simulink model "CM670A_HwAg1Meas"  (R2013b)
settings: Solver=FixedStepDiscrete  SolverMode=SingleTasking  StartTime=0.0  StopTime=22  FixedStep=0.002  RelTol=1e-3
values from neighbouring files (symbols this model uses):
  ELECGLBPRM_DEGPERREV_DEGPERREV_F32 = DataDict.Constant    [CM670A_HwAg1Meas_DataDict.m]
  ELECGLBPRM_HWAGCENTROFFS_HWDEG_F32 = DataDict.Constant    [CM670A_HwAg1Meas_DataDict.m]
  ELECGLBPRM_HWAGSATNLOWRLIM_HWDEG_F32 = DataDict.Constant    [CM670A_HwAg1Meas_DataDict.m]
  ELECGLBPRM_HWAGSATNUPPRLIM_HWDEG_F32 = DataDict.Constant    [CM670A_HwAg1Meas_DataDict.m]
  ELECGLBPRM_HWAGSCA_ULS_F32 = DataDict.Constant    [CM670A_HwAg1Meas_DataDict.m]
  ELECGLBPRM_HWAGSPURGEARRAT_ULS_F32 = DataDict.Constant    [CM670A_HwAg1Meas_DataDict.m]
  ELECGLBPRM_HWAGSPURTORINGGEARRATSNSR0_ULS_F32 = DataDict.Constant    [CM670A_HwAg1Meas_DataDict.m]
  ELECGLBPRM_HWAGSPURTORINGGEARRATSNSR1_ULS_F32 = DataDict.Constant    [CM670A_HwAg1Meas_DataDict.m]
  ELECGLBPRM_NOFLT_CNT_U08 = DataDict.Constant    [CM670A_HwAg1Meas_DataDict.m]
  ELECGLBPRM_OFFSTRIMNOTPRFMD_CNT_U08 = DataDict.Constant    [CM670A_HwAg1Meas_DataDict.m]
  ELECGLBPRM_PRTCLFLT_CNT_U08 = DataDict.Constant    [CM670A_HwAg1Meas_DataDict.m]
  ELECGLBPRM_SKIPSTEPFLT_CNT_U08 = DataDict.Constant    [CM670A_HwAg1Meas_DataDict.m]
  ELECGLBPRM_SNSRINTFLT_CNT_U08 = DataDict.Constant    [CM670A_HwAg1Meas_DataDict.m]
  ELECGLBPRM_VRNRERRFLT_CNT_U08 = DataDict.Constant    [CM670A_HwAg1Meas_DataDict.m]
  HWAG10THTOOTHTRIG_CNT_U08 = DataDict.ConfigParam    [CM670A_HwAg1Meas_DataDict.m]
  HWAG11THTOOTHTRIG_CNT_U08 = DataDict.ConfigParam    [CM670A_HwAg1Meas_DataDict.m]
  HwAg1IfFlt = DataDict.NTC    [CM670A_HwAg1Meas_DataDict.m]
  HwAg1MeasHwAg1IfFltFailStep = DataDict.Calibration    [CM670A_HwAg1Meas_DataDict.m]
  HwAg1MeasHwAg1IfFltPassStep = DataDict.Calibration    [CM670A_HwAg1Meas_DataDict.m]
  HwAg1MeasHwAg1Snsr0PrtclFltFailStep = DataDict.Calibration    [CM670A_HwAg1Meas_DataDict.m]
  HwAg1MeasHwAg1Snsr0PrtclFltPassStep = DataDict.Calibration    [CM670A_HwAg1Meas_DataDict.m]
  HwAg1MeasHwAg1Snsr1PrtclFltFailStep = DataDict.Calibration    [CM670A_HwAg1Meas_DataDict.m]
  HwAg1MeasHwAg1Snsr1PrtclFltPassStep = DataDict.Calibration    [CM670A_HwAg1Meas_DataDict.m]
  HwAg1MeasSnsr0Rev = DataDict.Calibration    [CM670A_HwAg1Meas_DataDict.m]
  HwAg1MeasSnsr1Rev = DataDict.Calibration    [CM670A_HwAg1Meas_DataDict.m]
  HwAg1MeasStep = DataDict.Calibration    [CM670A_HwAg1Meas_DataDict.m]
  HwAg1MeasVrnrErrThd = DataDict.Calibration    [CM670A_HwAg1Meas_DataDict.m]
  HwAg1MfgFlt = DataDict.NTC    [CM670A_HwAg1Meas_DataDict.m]
  HwAg1Snsr0PrtclFlt = DataDict.NTC    [CM670A_HwAg1Meas_DataDict.m]
  HwAg1Snsr1PrtclFlt = DataDict.NTC    [CM670A_HwAg1Meas_DataDict.m]
undefined symbols (not defined in the file or in its folder): NtcSts1, sigbuilder_block, SigQlfr1
libraries: simulink x30, NxtrNvM x3
(part 3 of 5)

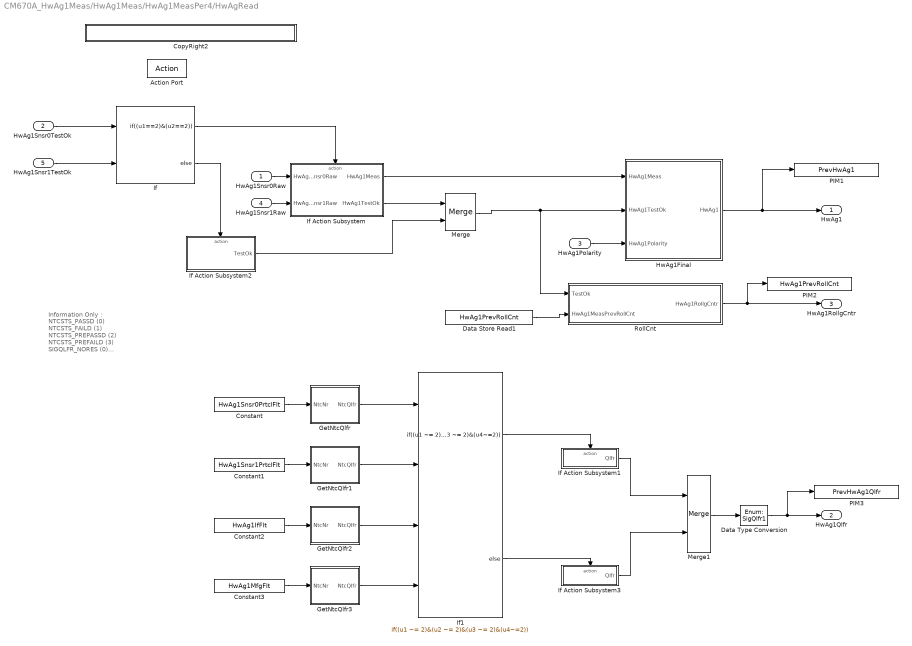
== system CM670A_HwAg1Meas/HwAg1Meas/HwAg1MeasPer4/HwAgRead ==
  note: Information Only :
      |
      | NTCSTS_PASSD            (0)
      | NTCSTS_FAILD              (1)
      | NTCSTS_PREPASSD    (2)
      | NTCSTS_PREFAILD      (3)
      |
      | SIGQLFR_NORES         (0)
      | SIGQLFR_PASSD          (1)
      | SIGQLFR_FAILD            (2)
  HwAg1Snsr0Raw : Inport
  HwAg1Snsr0TestOk : Inport  Port=2
  HwAg1Polarity : Inport  Port=3
  HwAg1Snsr1Raw : Inport  Port=4
  HwAg1Snsr1TestOk : Inport  Port=5
  Action Port : ActionPort  ActionType=then
  Constant : Constant  Value=HwAg1Snsr0PrtclFlt
  Constant1 : Constant  Value=HwAg1Snsr1PrtclFlt
  Constant2 : Constant  Value=HwAg1IfFlt
  Constant3 : Constant  Value=HwAg1MfgFlt
  CopyRight2 : Subsystem  Description=|  mask(Copyright Information){none=on}
      | Copyright info block.                                               
      |                                                                     
      | Place copyright information at the top of every subsystem in design.
      mask prompts: none "No parameters"
      mask help: Place copyright information at the top of every subsystem in design.
      mask Display:
      | NxtrConf = 'Nexteer Confidential';
      | 
      | sys = bdroot; %handle for the current model ("system")
      | first = get_param(sys,'Created');
      | first = first(end-3:end);  %year is last four digits
      | 
      | last = get_param(sys,'LastModifiedDate');
      | if isempty(last)
      |     last = datestr(now,'yyyy');
      | else
      |     last = last(end-3:end);
      | end
      | 
      | if strcmp(first,last)
      |     fprintf('%s -- Copyright %s Nexteer',NxtrConf,first)
      | else
      |     fprintf('%s -- %s%s- %s Nexteer',NxtrConf,char(169),first,last)
      | end
  Data Store Read1 : DataStoreRead  Priority=1  DataStoreName=HwAg1PrevRollCnt
  Data Type Conversion : DataTypeConversion  OutDataTypeStr=Enum: SigQlfr1
  GetNtcQlfr : Subsystem
  GetNtcQlfr1 : Subsystem
  GetNtcQlfr2 : Subsystem
  GetNtcQlfr3 : Subsystem
  HwAg1Final : Subsystem  RequirementInfo={'linktype_rmi_doors' '0000cf44 (/ESG Group/FDD Module Requirements/EA4 Specific/CM670A_HwAg1Meas)' '#CM670A_29' 'true' 'REQ: CM670A_29' '' ; 'linktype_rmi_doors' '0000cf44 (/ESG Group/FDD Module Requirements/EA4 Specific/CM670A_HwAg1Meas)' '#CM670A_32' 'true' 'REQ: CM670A_32' '' ; 'linktype_rmi_doors' '0000cf44 (/ESG Group/FDD Module Requirements/EA4 Specific/CM670A_HwAg1Meas)' '#CM670A_33' 'true' 'REQ: CM670A_33' '' } %GIDa_390fff4e_e0e4_4e0a_b1c2_f884cd2ad424
  If : If  NumInputs=2  IfExpression=(u1==2)&(u2==2)
  If Action Subsystem : Subsystem  TreatAsAtomicUnit=on
  If Action Subsystem1 : Subsystem  TreatAsAtomicUnit=on
  If Action Subsystem2 : Subsystem  TreatAsAtomicUnit=on
  If Action Subsystem3 : Subsystem  TreatAsAtomicUnit=on
  If1 : If  NumInputs=4  IfExpression=(u1 ~= 2)&(u2 ~= 2)&(u3 ~= 2)&(u4~=2)
  Merge : Merge
  Merge1 : Merge
  PIM1 : DataStoreWrite  RequirementInfo={} %GIDa_84bafa65_5fe1_4ee7_b90d_66bb4b4a2750  DataStoreName=PrevHwAg1
  PIM2 : DataStoreWrite  RequirementInfo={} %GIDa_617928b4_a9d1_4855_8092_551055b61714  Priority=2  DataStoreName=HwAg1PrevRollCnt
  PIM3 : DataStoreWrite  RequirementInfo={} %GIDa_3e11a627_fc39_44fa_9faf_fc285a087ff6  DataStoreName=PrevHwAg1Qlfr
  RollCnt : Stateflow chart  RequirementInfo={} %GIDa_3031df54_87b3_4189_88b6_56458e12ea75  TreatAsAtomicUnit=on
  HwAg1 : Outport  RequirementInfo={} %GIDa_c23b8355_c0ea_454a_a0f8_21e7eda4151f
  HwAg1Qlfr : Outport  RequirementInfo={'linktype_rmi_doors' '0000cf44 (/ESG Group/FDD Module Requirements/EA4 Specific/CM670A_HwAg1Meas)' '#CM670A_30' 'true' 'REQ: CM670A_30' '' } %GIDa_9c26b5fb_6b25_41c5_ba2e_96f197c0dca5  Port=2
  HwAg1RollgCntr : Outport  RequirementInfo={'linktype_rmi_doors' '0000cf44 (/ESG Group/FDD Module Requirements/EA4 Specific/CM670A_HwAg1Meas)' '#CM670A_31' 'true' 'REQ: CM670A_31' '' } %GIDa_eb7690db_9bf5_403e_b0dd_c189c54068be  Port=3
  wires:
  RollCnt/1(HwAg1RollgCntr) -> PIM2/1, HwAg1RollgCntr/1
  Constant/1 -> GetNtcQlfr/1(NtcNr)
  HwAg1Snsr0TestOk/1 -> If/1
  HwAg1Snsr1TestOk/1 -> If/2
  If/1 -> If Action Subsystem/Action
  If/2 -> If Action Subsystem2/Action
  If Action Subsystem2/1(TestOk) -> Merge/2
  If Action Subsystem/1(HwAg1Meas) -> HwAg1Final/1(HwAg1Meas)
  Constant1/1 -> GetNtcQlfr1/1(NtcNr)
  Constant2/1 -> GetNtcQlfr2/1(NtcNr)
  GetNtcQlfr/1(NtcQlfr) -> If1/1
  GetNtcQlfr1/1(NtcQlfr) -> If1/2
  GetNtcQlfr2/1(NtcQlfr) -> If1/3
  If1/1 -> If Action Subsystem1/Action
  If1/2 -> If Action Subsystem3/Action
  Merge1/1 -> Data Type Conversion/1
  If Action Subsystem1/1(Qlfr) -> Merge1/1
  If Action Subsystem3/1(Qlfr) -> Merge1/2
  If Action Subsystem/2(HwAg1TestOk) -> Merge/1
  HwAg1Polarity/1 -> HwAg1Final/3(HwAg1Polarity)
  GetNtcQlfr3/1(NtcQlfr) -> If1/4
  Constant3/1 -> GetNtcQlfr3/1(NtcNr)
  Merge/1 -> HwAg1Final/2(HwAg1TestOk), RollCnt/1(TestOk)
  HwAg1Final/1(HwAg1) -> PIM1/1, HwAg1/1
  HwAg1Snsr0Raw/1 -> If Action Subsystem/1(HwAg1Snsr0Raw)
  HwAg1Snsr1Raw/1 -> If Action Subsystem/2(HwAg1Snsr1Raw)
  Data Store Read1/1 -> RollCnt/2(HwAg1MeasPrevRollCnt)
  Data Type Conversion/1 -> PIM3/1, HwAg1Qlfr/1

== system CM670A_HwAg1Meas/HwAg1Meas/HwAg1MeasPer5/CopyRight2 ==

== system CM670A_HwAg1Meas/HwAg1Meas/HwAg1MeasPer5/If Action Subsystem ==
  Action Port : ActionPort  ActionType=then
  CopyRight2 : Subsystem  Description=|  mask(Copyright Information){none=on}
      | Copyright info block.                                               
      |                                                                     
      | Place copyright information at the top of every subsystem in design.
      mask prompts: none "No parameters"
      mask help: Place copyright information at the top of every subsystem in design.
      mask Display:
      | NxtrConf = 'Nexteer Confidential';
      | 
      | sys = bdroot; %handle for the current model ("system")
      | first = get_param(sys,'Created');
      | first = first(end-3:end);  %year is last four digits
      | 
      | last = get_param(sys,'LastModifiedDate');
      | if isempty(last)
      |     last = datestr(now,'yyyy');
      | else
      |     last = last(end-3:end);
      | end
      | 
      | if strcmp(first,last)
      |     fprintf('%s -- Copyright %s Nexteer',NxtrConf,first)
      | else
      |     fprintf('%s -- %s%s- %s Nexteer',NxtrConf,char(169),first,last)
      | end
  Data Type Conversion : DataTypeConversion  OutDataTypeStr=uint8
  NoFlt : Constant  RequirementInfo={} %GIDa_af25b43f_e757_49bd_94aa_be1229c5c8b6  Value=ELECGLBPRM_NOFLT_CNT_U08  OutDataTypeStr=uint8
  NtcSts : simulink/Sources/Enumerated Constant  OutDataTypeStr=Enum: NtcSts1  Value=NtcSts1.NTCSTS_PASSD  SampleTime=inf
  ParamByte : Outport
  TestOk : Outport  Port=2
  wires:
  NtcSts/1 -> Data Type Conversion/1
  NoFlt/1 -> ParamByte/1
  Data Type Conversion/1 -> TestOk/1

== system CM670A_HwAg1Meas/HwAg1Meas/HwAg1MeasPer5/If Action Subsystem1 ==
  Action Port : ActionPort  ActionType=else
  CopyRight2 : Subsystem  Description=|  mask(Copyright Information){none=on}
      | Copyright info block.                                               
      |                                                                     
      | Place copyright information at the top of every subsystem in design.
      mask prompts: none "No parameters"
      mask help: Place copyright information at the top of every subsystem in design.
      mask Display:
      | NxtrConf = 'Nexteer Confidential';
      | 
      | sys = bdroot; %handle for the current model ("system")
      | first = get_param(sys,'Created');
      | first = first(end-3:end);  %year is last four digits
      | 
      | last = get_param(sys,'LastModifiedDate');
      | if isempty(last)
      |     last = datestr(now,'yyyy');
      | else
      |     last = last(end-3:end);
      | end
      | 
      | if strcmp(first,last)
      |     fprintf('%s -- Copyright %s Nexteer',NxtrConf,first)
      | else
      |     fprintf('%s -- %s%s- %s Nexteer',NxtrConf,char(169),first,last)
      | end
  Data Type Conversion : DataTypeConversion  OutDataTypeStr=uint8
  NoFlt : Constant  RequirementInfo={} %GIDa_a79c1974_b7e9_4639_b05c_c7a17ce1d256  Value=ELECGLBPRM_OFFSTRIMNOTPRFMD_CNT_U08  OutDataTypeStr=uint8
  NtcSts : simulink/Sources/Enumerated Constant  OutDataTypeStr=Enum: NtcSts1  Value=NtcSts1.NTCSTS_FAILD  SampleTime=inf
  ParamByte : Outport
  TestOk : Outport  Port=2
  wires:
  NoFlt/1 -> ParamByte/1
  NtcSts/1 -> Data Type Conversion/1
  Data Type Conversion/1 -> TestOk/1

== system CM670A_HwAg1Meas/HwAg1Meas/HwAg1MeasPer5/SetNtcSts ==
  note: Note:
      |
      | - "ISO Fault Debounce Design" Simulink block intent to use here for Simulation purpose only. Do not Code this block
  NtcNr : Inport
  NtcStInfo : Inport  Port=2
  NtcSts : Inport  Port=3
  DebStep : Inport  Port=4
  CopyRight2 : Subsystem  Description=|  mask(Copyright Information){none=on}
      | Copyright info block.                                               
      |                                                                     
      | Place copyright information at the top of every subsystem in design.
      mask prompts: none "No parameters"
      mask help: Place copyright information at the top of every subsystem in design.
      mask Display:
      | NxtrConf = 'Nexteer Confidential';
      | 
      | sys = bdroot; %handle for the current model ("system")
      | first = get_param(sys,'Created');
      | first = first(end-3:end);  %year is last four digits
      | 
      | last = get_param(sys,'LastModifiedDate');
      | if isempty(last)
      |     last = datestr(now,'yyyy');
      | else
      |     last = last(end-3:end);
      | end
      | 
      | if strcmp(first,last)
      |     fprintf('%s -- Copyright %s Nexteer',NxtrConf,first)
      | else
      |     fprintf('%s -- %s%s- %s Nexteer',NxtrConf,char(169),first,last)
      | end
  Data Store Write : DataStoreWrite  DataStoreName=Ntc0X1FAQlfr
  Ground : Ground
  ISO Fault Debounce Design : Stateflow chart  TreatAsAtomicUnit=on
      settings: AttributesFormatString=|
      | Simulation Purpose Only.
      | Do Not Code this block
      | Diagnostic Manager Owns this requirement
  Scope1 : Scope  NumInputPorts=3
      settings: YMin=-5~-5~-5  YMax=5~5~5  SaveName=ScopeData5
  Terminator : Terminator
  Terminator1 : Terminator
  wires:
  Ground/1 -> ISO Fault Debounce Design/3(SvcClr)
  ISO Fault Debounce Design/1(Qualifier) -> Data Store Write/1, Scope1/3
  DebStep/1 -> Scope1/2, ISO Fault Debounce Design/2(DebStep)
  NtcSts/1 -> Scope1/1, ISO Fault Debounce Design/1(NtcSts)
  NtcNr/1 -> Terminator/1
  NtcStInfo/1 -> Terminator1/1

== system CM670A_HwAg1Meas/HwAg1Meas/HwAg1MeasInit1/GetRefTmr1MicroSec32bit/CopyRight2 ==

== system CM670A_HwAg1Meas/HwAg1Meas/HwAg1MeasInit1/GetTiSpan1MicroSec32bit/CopyRight2 ==

== system CM670A_HwAg1Meas/HwAg1Meas/HwAg1MeasInit1/IoHwAb_SetFctPrphlHwAg1/CopyRight2 ==

== system CM670A_HwAg1Meas/HwAg1Meas/HwAg1MeasPer1/GetRefTmr1MicroSec32bit1/CopyRight2 ==

== system CM670A_HwAg1Meas/HwAg1Meas/HwAg1MeasPer1/GetTiSpan1MicroSec32bit/CopyRight2 ==

== system CM670A_HwAg1Meas/HwAg1Meas/HwAg1MeasPer1/IncrementCount/CopyRight2 ==

== system CM670A_HwAg1Meas/HwAg1Meas/HwAg1MeasPer1/ResetCount/CopyRight2 ==

== system CM670A_HwAg1Meas/HwAg1Meas/HwAg1MeasPer2/Snsr0Read/CopyRight2 ==

== system CM670A_HwAg1Meas/HwAg1Meas/HwAg1MeasPer2/Snsr0Read/DebStepSelection ==
  TestOk : Inport
  CopyRight2 : Subsystem  Description=|  mask(Copyright Information){none=on}
      | Copyright info block.                                               
      |                                                                     
      | Place copyright information at the top of every subsystem in design.
      mask prompts: none "No parameters"
      mask help: Place copyright information at the top of every subsystem in design.
      mask Display:
      | NxtrConf = 'Nexteer Confidential';
      | 
      | sys = bdroot; %handle for the current model ("system")
      | first = get_param(sys,'Created');
      | first = first(end-3:end);  %year is last four digits
      | 
      | last = get_param(sys,'LastModifiedDate');
      | if isempty(last)
      |     last = datestr(now,'yyyy');
      | else
      |     last = last(end-3:end);
      | end
      | 
      | if strcmp(first,last)
      |     fprintf('%s -- Copyright %s Nexteer',NxtrConf,first)
      | else
      |     fprintf('%s -- %s%s- %s Nexteer',NxtrConf,char(169),first,last)
      | end
  NTCFailStepCal : Constant  Value=HwAg1MeasHwAg1Snsr0PrtclFltFailStep
  NTCPassStepCal : Constant  Value=HwAg1MeasHwAg1Snsr0PrtclFltPassStep
  Switch : Switch  Criteria=u2 > Threshold  Threshold=2
  DebStep : Outport  OutDataTypeStr=uint16
  wires:
  NTCFailStepCal/1 -> Switch/1
  Switch/1 -> DebStep/1
  NTCPassStepCal/1 -> Switch/3
  TestOk/1 -> Switch/2

== system CM670A_HwAg1Meas/HwAg1Meas/HwAg1MeasPer2/Snsr0Read/Do nothing ==
  Action Port : ActionPort  ActionType=else
  CopyRight2 : Subsystem  Description=|  mask(Copyright Information){none=on}
      | Copyright info block.                                               
      |                                                                     
      | Place copyright information at the top of every subsystem in design.
      mask prompts: none "No parameters"
      mask help: Place copyright information at the top of every subsystem in design.
      mask Display:
      | NxtrConf = 'Nexteer Confidential';
      | 
      | sys = bdroot; %handle for the current model ("system")
      | first = get_param(sys,'Created');
      | first = first(end-3:end);  %year is last four digits
      | 
      | last = get_param(sys,'LastModifiedDate');
      | if isempty(last)
      |     last = datestr(now,'yyyy');
      | else
      |     last = last(end-3:end);
      | end
      | 
      | if strcmp(first,last)
      |     fprintf('%s -- Copyright %s Nexteer',NxtrConf,first)
      | else
      |     fprintf('%s -- %s%s- %s Nexteer',NxtrConf,char(169),first,last)
      | end

== system CM670A_HwAg1Meas/HwAg1Meas/HwAg1MeasPer2/Snsr0Read/RawHwAgRead ==
  Snsr0CS : Inport
  Snsr0FRS : Inport  Port=2
  Snsr0FCCN : Inport  Port=3
  Snsr0Data : Inport  Port=4
  Snsr0Id : Inport  Port=5
  Bus Selector : BusSelector  OutputSignals=RawHwAg,TestOk,ParamByte
  Bus Selector1 : BusSelector  OutputSignals=RawHwAg,TestOk,ParamByte
  CopyRight2 : Subsystem  Description=|  mask(Copyright Information){none=on}
      | Copyright info block.                                               
      |                                                                     
      | Place copyright information at the top of every subsystem in design.
      mask prompts: none "No parameters"
      mask help: Place copyright information at the top of every subsystem in design.
      mask Display:
      | NxtrConf = 'Nexteer Confidential';
      | 
      | sys = bdroot; %handle for the current model ("system")
      | first = get_param(sys,'Created');
      | first = first(end-3:end);  %year is last four digits
      | 
      | last = get_param(sys,'LastModifiedDate');
      | if isempty(last)
      |     last = datestr(now,'yyyy');
      | else
      |     last = last(end-3:end);
      | end
      | 
      | if strcmp(first,last)
      |     fprintf('%s -- Copyright %s Nexteer',NxtrConf,first)
      | else
      |     fprintf('%s -- %s%s- %s Nexteer',NxtrConf,char(169),first,last)
      | end
  If : If  RequirementInfo={} %GIDa_2f644cf5_4c0f_42f4_aa5e_d14eb49d3684  IfExpression=u1 ~= 0
  Merge : Merge
  Merge1 : Merge
  Merge2 : Merge
  NewMsg : Subsystem  TreatAsAtomicUnit=on
  NoNewMsg : Subsystem  RequirementInfo={'linktype_rmi_doors' '0000cf44 (/ESG Group/FDD Module Requirements/EA4 Specific/CM670A_HwAg1Meas)' '#CM670A_47' 'true' 'REQ: CM670A_47' '' } %GIDa_69e0972d_6120_427f_87c3_f6166b66255c  TreatAsAtomicUnit=on
      mask Display: disp('NoNewMsg')
  Snsr0Scope : Scope  NumInputPorts=3
      settings: TimeRange=10  YMin=0~1.5~-0.5  YMax=5000~3.5~4.5
  RawHwAg : Outport
  TestOk : Outport  Port=2
  ParamByte : Outport  Port=3
  wires:
  If/1 -> NewMsg/Action  "NoFault"
  If/2 -> NoNewMsg/Action  "Fault"
  NewMsg/1(Out1) -> Bus Selector/1
  NoNewMsg/1(Out1) -> Bus Selector1/1
  Bus Selector1/1 -> Merge2/1  "<RawHwAg>"
  Bus Selector/1 -> Merge2/2  "<RawHwAg>"
  Bus Selector1/2 -> Merge/1  "<TestOk>"
  Bus Selector/2 -> Merge/2  "<TestOk>"
  Bus Selector1/3 -> Merge1/1  "<ParamByte>"
  Bus Selector/3 -> Merge1/2  "<ParamByte>"
  Merge2/1 -> RawHwAg/1, Snsr0Scope/1  "RawHwAg"
  Merge/1 -> Snsr0Scope/2, TestOk/1  "TestOk"
  Merge1/1 -> Snsr0Scope/3, ParamByte/1  "ParamByte"
  Snsr0FRS/1 -> If/1
  Snsr0CS/1 -> NewMsg/1(Snsr0CS)
  Snsr0FCCN/1 -> NewMsg/2(Snsr0FCCN)
  Snsr0Data/1 -> NewMsg/4(Snsr0Data)
  Snsr0Id/1 -> NewMsg/3(Snsr0Id)

== system CM670A_HwAg1Meas/HwAg1Meas/HwAg1MeasPer2/Snsr0Read/Read the Flag ==
  RegInpRSENT2FND : Inport
  Action Port : ActionPort  ActionType=then
  CopyRight2 : Subsystem  Description=|  mask(Copyright Information){none=on}
      | Copyright info block.                                               
      |                                                                     
      | Place copyright information at the top of every subsystem in design.
      mask prompts: none "No parameters"
      mask help: Place copyright information at the top of every subsystem in design.
      mask Display:
      | NxtrConf = 'Nexteer Confidential';
      | 
      | sys = bdroot; %handle for the current model ("system")
      | first = get_param(sys,'Created');
      | first = first(end-3:end);  %year is last four digits
      | 
      | last = get_param(sys,'LastModifiedDate');
      | if isempty(last)
      |     last = datestr(now,'yyyy');
      | else
      |     last = last(end-3:end);
      | end
      | 
      | if strcmp(first,last)
      |     fprintf('%s -- Copyright %s Nexteer',NxtrConf,first)
      | else
      |     fprintf('%s -- %s%s- %s Nexteer',NxtrConf,char(169),first,last)
      | end
  RSENT2DummyRead : Terminator
  wires:
  RegInpRSENT2FND/1 -> RSENT2DummyRead/1

== system CM670A_HwAg1Meas/HwAg1Meas/HwAg1MeasPer2/Snsr0Read/SetNtcSts ==
  note: Note:
      |
      | - "ISO Fault Debounce Design" Simulink block intent to use here for Simulation purpose only. Do not Code this block
  NtcNr : Inport
  NtcStInfo : Inport  Port=2
  NtcSts : Inport  Port=3
  DebStep : Inport  Port=4
  CopyRight2 : Subsystem  Description=|  mask(Copyright Information){none=on}
      | Copyright info block.                                               
      |                                                                     
      | Place copyright information at the top of every subsystem in design.
      mask prompts: none "No parameters"
      mask help: Place copyright information at the top of every subsystem in design.
      mask Display:
      | NxtrConf = 'Nexteer Confidential';
      | 
      | sys = bdroot; %handle for the current model ("system")
      | first = get_param(sys,'Created');
      | first = first(end-3:end);  %year is last four digits
      | 
      | last = get_param(sys,'LastModifiedDate');
      | if isempty(last)
      |     last = datestr(now,'yyyy');
      | else
      |     last = last(end-3:end);
      | end
      | 
      | if strcmp(first,last)
      |     fprintf('%s -- Copyright %s Nexteer',NxtrConf,first)
      | else
      |     fprintf('%s -- %s%s- %s Nexteer',NxtrConf,char(169),first,last)
      | end
  Data Store Write : DataStoreWrite  DataStoreName=Ntc0x097Qlfr
  Ground : Ground
  ISO Fault Debounce Design : Stateflow chart  TreatAsAtomicUnit=on
      settings: AttributesFormatString=|
      | Simulation Purpose Only.
      | Do Not Code this block
      | Diagnostic Manager Owns this requirement
  Scope1 : Scope  NumInputPorts=3
      settings: YMin=-5~-5~-5  YMax=5~5~5  SaveName=ScopeData5
  Terminator : Terminator
  Terminator1 : Terminator
  wires:
  Ground/1 -> ISO Fault Debounce Design/3(SvcClr)
  ISO Fault Debounce Design/1(Qualifier) -> Data Store Write/1, Scope1/3
  DebStep/1 -> Scope1/2, ISO Fault Debounce Design/2(DebStep)
  NtcSts/1 -> Scope1/1, ISO Fault Debounce Design/1(NtcSts)
  NtcNr/1 -> Terminator/1
  NtcStInfo/1 -> Terminator1/1

== system CM670A_HwAg1Meas/HwAg1Meas/HwAg1MeasPer2/Snsr0Read1/CopyRight2 ==

== system CM670A_HwAg1Meas/HwAg1Meas/HwAg1MeasPer3/Snsr1Read/CopyRight2 ==

== system CM670A_HwAg1Meas/HwAg1Meas/HwAg1MeasPer3/Snsr1Read/DebStepSelection ==
  TestOk : Inport
  CopyRight2 : Subsystem  Description=|  mask(Copyright Information){none=on}
      | Copyright info block.                                               
      |                                                                     
      | Place copyright information at the top of every subsystem in design.
      mask prompts: none "No parameters"
      mask help: Place copyright information at the top of every subsystem in design.
      mask Display:
      | NxtrConf = 'Nexteer Confidential';
      | 
      | sys = bdroot; %handle for the current model ("system")
      | first = get_param(sys,'Created');
      | first = first(end-3:end);  %year is last four digits
      | 
      | last = get_param(sys,'LastModifiedDate');
      | if isempty(last)
      |     last = datestr(now,'yyyy');
      | else
      |     last = last(end-3:end);
      | end
      | 
      | if strcmp(first,last)
      |     fprintf('%s -- Copyright %s Nexteer',NxtrConf,first)
      | else
      |     fprintf('%s -- %s%s- %s Nexteer',NxtrConf,char(169),first,last)
      | end
  NTCFailStepCal : Constant  Value=HwAg1MeasHwAg1Snsr1PrtclFltFailStep
  NTCPassStepCal : Constant  Value=HwAg1MeasHwAg1Snsr1PrtclFltPassStep
  Switch : Switch  Criteria=u2 > Threshold  Threshold=2
  DebStep : Outport  OutDataTypeStr=uint16
  wires:
  NTCFailStepCal/1 -> Switch/1
  Switch/1 -> DebStep/1
  NTCPassStepCal/1 -> Switch/3
  TestOk/1 -> Switch/2

== system CM670A_HwAg1Meas/HwAg1Meas/HwAg1MeasPer3/Snsr1Read/Do nothing ==
  Action Port : ActionPort  ActionType=else
  CopyRight2 : Subsystem  Description=|  mask(Copyright Information){none=on}
      | Copyright info block.                                               
      |                                                                     
      | Place copyright information at the top of every subsystem in design.
      mask prompts: none "No parameters"
      mask help: Place copyright information at the top of every subsystem in design.
      mask Display:
      | NxtrConf = 'Nexteer Confidential';
      | 
      | sys = bdroot; %handle for the current model ("system")
      | first = get_param(sys,'Created');
      | first = first(end-3:end);  %year is last four digits
      | 
      | last = get_param(sys,'LastModifiedDate');
      | if isempty(last)
      |     last = datestr(now,'yyyy');
      | else
      |     last = last(end-3:end);
      | end
      | 
      | if strcmp(first,last)
      |     fprintf('%s -- Copyright %s Nexteer',NxtrConf,first)
      | else
      |     fprintf('%s -- %s%s- %s Nexteer',NxtrConf,char(169),first,last)
      | end

== system CM670A_HwAg1Meas/HwAg1Meas/HwAg1MeasPer3/Snsr1Read/Do nothing1 ==
  Action Port : ActionPort  ActionType=else
  CopyRight2 : Subsystem  Description=|  mask(Copyright Information){none=on}
      | Copyright info block.                                               
      |                                                                     
      | Place copyright information at the top of every subsystem in design.
      mask prompts: none "No parameters"
      mask help: Place copyright information at the top of every subsystem in design.
      mask Display:
      | NxtrConf = 'Nexteer Confidential';
      | 
      | sys = bdroot; %handle for the current model ("system")
      | first = get_param(sys,'Created');
      | first = first(end-3:end);  %year is last four digits
      | 
      | last = get_param(sys,'LastModifiedDate');
      | if isempty(last)
      |     last = datestr(now,'yyyy');
      | else
      |     last = last(end-3:end);
      | end
      | 
      | if strcmp(first,last)
      |     fprintf('%s -- Copyright %s Nexteer',NxtrConf,first)
      | else
      |     fprintf('%s -- %s%s- %s Nexteer',NxtrConf,char(169),first,last)
      | end

== system CM670A_HwAg1Meas/HwAg1Meas/HwAg1MeasPer3/Snsr1Read/RawHwAgRead ==
  Snsr1CS : Inport
  Snsr1FRS : Inport  Port=2
  Snsr1FCCN : Inport  Port=3
  Snsr1Data : Inport  Port=4
  Snsr1Id : Inport  Port=5
  Bus Selector : BusSelector  OutputSignals=RawHwAg,TestOk,ParamByte
  Bus Selector1 : BusSelector  OutputSignals=RawHwAg,TestOk,ParamByte
  CopyRight2 : Subsystem  Description=|  mask(Copyright Information){none=on}
      | Copyright info block.                                               
      |                                                                     
      | Place copyright information at the top of every subsystem in design.
      mask prompts: none "No parameters"
      mask help: Place copyright information at the top of every subsystem in design.
      mask Display:
      | NxtrConf = 'Nexteer Confidential';
      | 
      | sys = bdroot; %handle for the current model ("system")
      | first = get_param(sys,'Created');
      | first = first(end-3:end);  %year is last four digits
      | 
      | last = get_param(sys,'LastModifiedDate');
      | if isempty(last)
      |     last = datestr(now,'yyyy');
      | else
      |     last = last(end-3:end);
      | end
      | 
      | if strcmp(first,last)
      |     fprintf('%s -- Copyright %s Nexteer',NxtrConf,first)
      | else
      |     fprintf('%s -- %s%s- %s Nexteer',NxtrConf,char(169),first,last)
      | end
  If : If  RequirementInfo={} %GIDa_15f483e9_befa_45a2_b74e_1f3bb1cc8902  IfExpression=u1 ~= 0
  Merge : Merge
  Merge1 : Merge
  Merge2 : Merge
  NewMsg : Subsystem  TreatAsAtomicUnit=on
  NoNewMsg : Subsystem  RequirementInfo={'linktype_rmi_doors' '0000cf44 (/ESG Group/FDD Module Requirements/EA4 Specific/CM670A_HwAg1Meas)' '#CM670A_70' 'true' 'REQ: CM670A_70' '' } %GIDa_121b31c2_4ce6_4121_b66f_436f1ca411f9  TreatAsAtomicUnit=on
      mask Display: disp('NoNewMsg')
  Snsr0Scope : Scope  NumInputPorts=3
      settings: TimeRange=10  YMin=0~2~7.6  YMax=4250~2~8.4
  RawHwAg : Outport
  TestOk : Outport  Port=2
  ParamByte : Outport  Port=3
  wires:
  If/1 -> NewMsg/Action  "NoFault"
  If/2 -> NoNewMsg/Action  "Fault"
  NewMsg/1(Out1) -> Bus Selector/1
  NoNewMsg/1(Out1) -> Bus Selector1/1
  Bus Selector1/1 -> Merge2/1  "<RawHwAg>"
  Bus Selector/1 -> Merge2/2  "<RawHwAg>"
  Bus Selector1/2 -> Merge/1  "<TestOk>"
  Bus Selector/2 -> Merge/2  "<TestOk>"
  Bus Selector1/3 -> Merge1/1  "<ParamByte>"
  Bus Selector/3 -> Merge1/2  "<ParamByte>"
  Merge2/1 -> RawHwAg/1, Snsr0Scope/1  "RawHwAg"
  Merge/1 -> Snsr0Scope/2, TestOk/1  "TestOk"
  Merge1/1 -> Snsr0Scope/3, ParamByte/1  "ParamByte"
  Snsr1FRS/1 -> If/1
  Snsr1CS/1 -> NewMsg/1(Snsr1CS)
  Snsr1FCCN/1 -> NewMsg/2(Snsr1FCCN)
  Snsr1Data/1 -> NewMsg/4(Snsr1Data)
  Snsr1Id/1 -> NewMsg/3(Snsr1Id)

== system CM670A_HwAg1Meas/HwAg1Meas/HwAg1MeasPer3/Snsr1Read/Read the Flag ==
  RegInpRSENT2FND : Inport
  Action Port : ActionPort  ActionType=then
  CopyRight2 : Subsystem  Description=|  mask(Copyright Information){none=on}
      | Copyright info block.                                               
      |                                                                     
      | Place copyright information at the top of every subsystem in design.
      mask prompts: none "No parameters"
      mask help: Place copyright information at the top of every subsystem in design.
      mask Display:
      | NxtrConf = 'Nexteer Confidential';
      | 
      | sys = bdroot; %handle for the current model ("system")
      | first = get_param(sys,'Created');
      | first = first(end-3:end);  %year is last four digits
      | 
      | last = get_param(sys,'LastModifiedDate');
      | if isempty(last)
      |     last = datestr(now,'yyyy');
      | else
      |     last = last(end-3:end);
      | end
      | 
      | if strcmp(first,last)
      |     fprintf('%s -- Copyright %s Nexteer',NxtrConf,first)
      | else
      |     fprintf('%s -- %s%s- %s Nexteer',NxtrConf,char(169),first,last)
      | end
  RSENT2DummyRead : Terminator
  wires:
  RegInpRSENT2FND/1 -> RSENT2DummyRead/1

== system CM670A_HwAg1Meas/HwAg1Meas/HwAg1MeasPer3/Snsr1Read/SetNtcSts ==
  note: Note:
      |
      | - "ISO Fault Debounce Design" Simulink block intent to use here for Simulation purpose only. Do not Code this block
  NtcNr : Inport
  NtcStInfo : Inport  Port=2
  NtcSts : Inport  Port=3
  DebStep : Inport  Port=4
  CopyRight2 : Subsystem  Description=|  mask(Copyright Information){none=on}
      | Copyright info block.                                               
      |                                                                     
      | Place copyright information at the top of every subsystem in design.
      mask prompts: none "No parameters"
      mask help: Place copyright information at the top of every subsystem in design.
      mask Display:
      | NxtrConf = 'Nexteer Confidential';
      | 
      | sys = bdroot; %handle for the current model ("system")
      | first = get_param(sys,'Created');
      | first = first(end-3:end);  %year is last four digits
      | 
      | last = get_param(sys,'LastModifiedDate');
      | if isempty(last)
      |     last = datestr(now,'yyyy');
      | else
      |     last = last(end-3:end);
      | end
      | 
      | if strcmp(first,last)
      |     fprintf('%s -- Copyright %s Nexteer',NxtrConf,first)
      | else
      |     fprintf('%s -- %s%s- %s Nexteer',NxtrConf,char(169),first,last)
      | end
  Data Store Write : DataStoreWrite  DataStoreName=Ntc0x099Qlfr
  Ground : Ground
  ISO Fault Debounce Design : Stateflow chart  TreatAsAtomicUnit=on
      settings: AttributesFormatString=|
      | Simulation Purpose Only.
      | Do Not Code this block
      | Diagnostic Manager Owns this requirement
  Scope1 : Scope  NumInputPorts=3
      settings: YMin=-5~-5~-5  YMax=5~5~5  SaveName=ScopeData5
  Terminator : Terminator
  Terminator1 : Terminator
  wires:
  Ground/1 -> ISO Fault Debounce Design/3(SvcClr)
  ISO Fault Debounce Design/1(Qualifier) -> Data Store Write/1, Scope1/3
  DebStep/1 -> Scope1/2, ISO Fault Debounce Design/2(DebStep)
  NtcSts/1 -> Scope1/1, ISO Fault Debounce Design/1(NtcSts)
  NtcNr/1 -> Terminator/1
  NtcStInfo/1 -> Terminator1/1

== system CM670A_HwAg1Meas/HwAg1Meas/HwAg1MeasPer3/Snsr1Read/SyncPulse ==
  note: Information only:
      |
      | - Sensors are synchronized if they receive 104us tick wide SPCT low pulse.
  note: Follow below steps in same order:
      |
      | 1. Send Sensor Synchronization command Pulse (RegOutRSENT2SPCT = 103U)
      | 1a. asm"syncm"
      | 2. NRS Flag Check: If the flag (RegInpRSENT2NRS==1) is Set Clear the flag RegOutRSENT2NRC=1
      | 2a. 2us wait timer
      | 3. Execute RegOutRSENT2SPCT = 103U
  RegInpRSENT2NRS : Inport
  Action Port : ActionPort  ActionType=then
  CopyRight2 : Subsystem  Description=|  mask(Copyright Information){none=on}
      | Copyright info block.                                               
      |                                                                     
      | Place copyright information at the top of every subsystem in design.
      mask prompts: none "No parameters"
      mask help: Place copyright information at the top of every subsystem in design.
      mask Display:
      | NxtrConf = 'Nexteer Confidential';
      | 
      | sys = bdroot; %handle for the current model ("system")
      | first = get_param(sys,'Created');
      | first = first(end-3:end);  %year is last four digits
      | 
      | last = get_param(sys,'LastModifiedDate');
      | if isempty(last)
      |     last = datestr(now,'yyyy');
      | else
      |     last = last(end-3:end);
      | end
      | 
      | if strcmp(first,last)
      |     fprintf('%s -- Copyright %s Nexteer',NxtrConf,first)
      | else
      |     fprintf('%s -- %s%s- %s Nexteer',NxtrConf,char(169),first,last)
      | end
  GetRefTmr1MicroSec32bit : Subsystem
      settings: AttributesFormatString=Client Call : Start Time
  GetTiSpan1MicroSec32bit : Subsystem
  Ground : Ground
  Ground3 : Ground
  Terminator : Terminator
  Terminator1 : Terminator
  RegOutRSENT2SPCT : Outport
  RegOutRSENT2NRC : Outport  Port=2
  wires:
  RegInpRSENT2NRS/1 -> Terminator/1
  Ground/1 -> RegOutRSENT2SPCT/1
  GetTiSpan1MicroSec32bit/1(TiSpan) -> Terminator1/1
  GetRefTmr1MicroSec32bit/1(RefTmr) -> GetTiSpan1MicroSec32bit/1(RefTmr)
  Ground3/1 -> RegOutRSENT2NRC/1

== system CM670A_HwAg1Meas/HwAg1Meas/HwAg1MeasPer3/Snsr1Read1/CopyRight2 ==

== system CM670A_HwAg1Meas/HwAg1Meas/HwAg1MeasPer4/HwAgPrevRead/CopyRight2 ==

== system CM670A_HwAg1Meas/HwAg1Meas/HwAg1MeasPer4/HwAgRead/CopyRight2 ==

== system CM670A_HwAg1Meas/HwAg1Meas/HwAg1MeasPer4/HwAgRead/GetNtcQlfr ==
  NtcNr : Inport
  CopyRight2 : Subsystem  Description=|  mask(Copyright Information){none=on}
      | Copyright info block.                                               
      |                                                                     
      | Place copyright information at the top of every subsystem in design.
      mask prompts: none "No parameters"
      mask help: Place copyright information at the top of every subsystem in design.
      mask Display:
      | NxtrConf = 'Nexteer Confidential';
      | 
      | sys = bdroot; %handle for the current model ("system")
      | first = get_param(sys,'Created');
      | first = first(end-3:end);  %year is last four digits
      | 
      | last = get_param(sys,'LastModifiedDate');
      | if isempty(last)
      |     last = datestr(now,'yyyy');
      | else
      |     last = last(end-3:end);
      | end
      | 
      | if strcmp(first,last)
      |     fprintf('%s -- Copyright %s Nexteer',NxtrConf,first)
      | else
      |     fprintf('%s -- %s%s- %s Nexteer',NxtrConf,char(169),first,last)
      | end
  Data Store Read : DataStoreRead  DataStoreName=Ntc0x097Qlfr
  Terminator : Terminator
  NtcQlfr : Outport
  wires:
  Data Store Read/1 -> NtcQlfr/1
  NtcNr/1 -> Terminator/1

== system CM670A_HwAg1Meas/HwAg1Meas/HwAg1MeasPer4/HwAgRead/GetNtcQlfr1 ==
  NtcNr : Inport
  CopyRight2 : Subsystem  Description=|  mask(Copyright Information){none=on}
      | Copyright info block.                                               
      |                                                                     
      | Place copyright information at the top of every subsystem in design.
      mask prompts: none "No parameters"
      mask help: Place copyright information at the top of every subsystem in design.
      mask Display:
      | NxtrConf = 'Nexteer Confidential';
      | 
      | sys = bdroot; %handle for the current model ("system")
      | first = get_param(sys,'Created');
      | first = first(end-3:end);  %year is last four digits
      | 
      | last = get_param(sys,'LastModifiedDate');
      | if isempty(last)
      |     last = datestr(now,'yyyy');
      | else
      |     last = last(end-3:end);
      | end
      | 
      | if strcmp(first,last)
      |     fprintf('%s -- Copyright %s Nexteer',NxtrConf,first)
      | else
      |     fprintf('%s -- %s%s- %s Nexteer',NxtrConf,char(169),first,last)
      | end
  Data Store Read : DataStoreRead  DataStoreName=Ntc0x099Qlfr
  Terminator : Terminator
  NtcQlfr : Outport
  wires:
  Data Store Read/1 -> NtcQlfr/1
  NtcNr/1 -> Terminator/1

== system CM670A_HwAg1Meas/HwAg1Meas/HwAg1MeasPer4/HwAgRead/GetNtcQlfr2 ==
  NtcNr : Inport
  CopyRight2 : Subsystem  Description=|  mask(Copyright Information){none=on}
      | Copyright info block.                                               
      |                                                                     
      | Place copyright information at the top of every subsystem in design.
      mask prompts: none "No parameters"
      mask help: Place copyright information at the top of every subsystem in design.
      mask Display:
      | NxtrConf = 'Nexteer Confidential';
      | 
      | sys = bdroot; %handle for the current model ("system")
      | first = get_param(sys,'Created');
      | first = first(end-3:end);  %year is last four digits
      | 
      | last = get_param(sys,'LastModifiedDate');
      | if isempty(last)
      |     last = datestr(now,'yyyy');
      | else
      |     last = last(end-3:end);
      | end
      | 
      | if strcmp(first,last)
      |     fprintf('%s -- Copyright %s Nexteer',NxtrConf,first)
      | else
      |     fprintf('%s -- %s%s- %s Nexteer',NxtrConf,char(169),first,last)
      | end
  Data Store Read : DataStoreRead  DataStoreName=Ntc0x098Qlfr
  Terminator : Terminator
  NtcQlfr : Outport
  wires:
  Data Store Read/1 -> NtcQlfr/1
  NtcNr/1 -> Terminator/1

== system CM670A_HwAg1Meas/HwAg1Meas/HwAg1MeasPer4/HwAgRead/GetNtcQlfr3 ==
  NtcNr : Inport
  CopyRight2 : Subsystem  Description=|  mask(Copyright Information){none=on}
      | Copyright info block.                                               
      |                                                                     
      | Place copyright information at the top of every subsystem in design.
      mask prompts: none "No parameters"
      mask help: Place copyright information at the top of every subsystem in design.
      mask Display:
      | NxtrConf = 'Nexteer Confidential';
      | 
      | sys = bdroot; %handle for the current model ("system")
      | first = get_param(sys,'Created');
      | first = first(end-3:end);  %year is last four digits
      | 
      | last = get_param(sys,'LastModifiedDate');
      | if isempty(last)
      |     last = datestr(now,'yyyy');
      | else
      |     last = last(end-3:end);
      | end
      | 
      | if strcmp(first,last)
      |     fprintf('%s -- Copyright %s Nexteer',NxtrConf,first)
      | else
      |     fprintf('%s -- %s%s- %s Nexteer',NxtrConf,char(169),first,last)
      | end
  Data Store Read : DataStoreRead  DataStoreName=Ntc0X1FAQlfr
  Terminator : Terminator
  NtcQlfr : Outport
  wires:
  Data Store Read/1 -> NtcQlfr/1
  NtcNr/1 -> Terminator/1

== system CM670A_HwAg1Meas/HwAg1Meas/HwAg1MeasPer4/HwAgRead/HwAg1Final ==
  HwAg1Meas : Inport  OutDataTypeStr=single
  HwAg1TestOk : Inport  Port=2
  HwAg1Polarity : Inport  Port=3
  CopyRight2 : Subsystem  Description=|  mask(Copyright Information){none=on}
      | Copyright info block.                                               
      |                                                                     
      | Place copyright information at the top of every subsystem in design.
      mask prompts: none "No parameters"
      mask help: Place copyright information at the top of every subsystem in design.
      mask Display:
      | NxtrConf = 'Nexteer Confidential';
      | 
      | sys = bdroot; %handle for the current model ("system")
      | first = get_param(sys,'Created');
      | first = first(end-3:end);  %year is last four digits
      | 
      | last = get_param(sys,'LastModifiedDate');
      | if isempty(last)
      |     last = datestr(now,'yyyy');
      | else
      |     last = last(end-3:end);
      | end
      | 
      | if strcmp(first,last)
      |     fprintf('%s -- Copyright %s Nexteer',NxtrConf,first)
      | else
      |     fprintf('%s -- %s%s- %s Nexteer',NxtrConf,char(169),first,last)
      | end
  ModRoll : Stateflow chart  RequirementInfo={} %GIDa_8cd37f12_0bd5_4979_8512_84bca554322a  TreatAsAtomicUnit=on
  NVM Shadow RAM : DataStoreRead  DataStoreName=HwAg1OffsTrim
  PIM : DataStoreWrite  RequirementInfo={'linktype_rmi_doors' '0000cf44 (/ESG Group/FDD Module Requirements/EA4 Specific/CM670A_HwAg1Meas)' '#CM670A_50' 'true' 'REQ: CM670A_50' '' } %GIDa_df40a191_3229_49ea_ae94_e8070f81128a  DataStoreName=HwAg1PrevHwAg1
  PIM1 : DataStoreRead  DataStoreName=HwAg1PrevHwAg1
  Product : Product
  Saturation1 : Saturate  UpperLimit=ELECGLBPRM_HWAGSATNUPPRLIM_HWDEG_F32  LowerLimit=ELECGLBPRM_HWAGSATNLOWRLIM_HWDEG_F32
  Subtract1 : Sum  Inputs=+-
  Switch : Switch  Criteria=u2 > Threshold  Threshold=2
  HwAg1 : Outport  RequirementInfo={'linktype_rmi_doors' '0000cf44 (/ESG Group/FDD Module Requirements/EA4 Specific/CM670A_HwAg1Meas)' '#CM670A_26' 'true' 'REQ: CM670A_26' '' } %GIDa_5a806761_ebcc_4d88_9266_ae7fea8466ec
  wires:
  Product/1 -> Switch/3
  Switch/1 -> PIM/1, Subtract1/1
  HwAg1TestOk/1 -> Switch/2
  HwAg1Meas/1 -> Product/1
  HwAg1Polarity/1 -> Product/2
  NVM Shadow RAM/1 -> Subtract1/2
  PIM1/1 -> Switch/1
  ModRoll/1(OutVal) -> Saturation1/1
  Subtract1/1 -> ModRoll/1(RawVal)
  Saturation1/1 -> HwAg1/1

== system CM670A_HwAg1Meas/HwAg1Meas/HwAg1MeasPer4/HwAgRead/If Action Subsystem ==
  note: Information only:
      |
      | - AbsoluteHandWheel Angle Calculation
  HwAg1Snsr0Raw : Inport
  HwAg1Snsr1Raw : Inport  Port=2
  Action Port : ActionPort  PropagateVarSize=During execution  ActionType=then
  AdjStepCalc : Subsystem
  Constant : Constant  Value=HwAg1IfFlt
  CopyRight2 : Subsystem  Description=|  mask(Copyright Information){none=on}
      | Copyright info block.                                               
      |                                                                     
      | Place copyright information at the top of every subsystem in design.
      mask prompts: none "No parameters"
      mask help: Place copyright information at the top of every subsystem in design.
      mask Display:
      | NxtrConf = 'Nexteer Confidential';
      | 
      | sys = bdroot; %handle for the current model ("system")
      | first = get_param(sys,'Created');
      | first = first(end-3:end);  %year is last four digits
      | 
      | last = get_param(sys,'LastModifiedDate');
      | if isempty(last)
      |     last = datestr(now,'yyyy');
      | else
      |     last = last(end-3:end);
      | end
      | 
      | if strcmp(first,last)
      |     fprintf('%s -- Copyright %s Nexteer',NxtrConf,first)
      | else
      |     fprintf('%s -- %s%s- %s Nexteer',NxtrConf,char(169),first,last)
      | end
  DebStepSelection : Subsystem
  HwAg1Snsr0RelCalc : Subsystem
  HwAg1Snsr1RelCalc : Subsystem
  SetNtcSts : Subsystem  RequirementInfo={'linktype_rmi_doors' '0000cf44 (/ESG Group/FDD Module Requirements/EA4 Specific/CM670A_HwAg1Meas)' '#CM670A_93' 'true' 'REQ: CM670A_93' '' } %GIDa_efc373e6_c473_4227_a98a_36ef015df3b4
  HwAg1Meas : Outport
  HwAg1TestOk : Outport  Port=2
  wires:
  HwAg1Snsr0Raw/1 -> HwAg1Snsr0RelCalc/1(RawHwAg1Snsr0)
  HwAg1Snsr1Raw/1 -> HwAg1Snsr1RelCalc/1(RawHwAg1Snsr1)
  HwAg1Snsr1RelCalc/1(HwAg1Snsr1Rel) -> AdjStepCalc/2(HwAg1Sns1Rel)
  HwAg1Snsr0RelCalc/1(HwAg1Snsr0Rel) -> AdjStepCalc/1(HwAg1Snsr0Rel)
  AdjStepCalc/1(HwAg1) -> HwAg1Meas/1
  DebStepSelection/1(DebStep) -> SetNtcSts/4(DebStep)
  Constant/1 -> SetNtcSts/1(NtcNr)  "NtcNr"
  AdjStepCalc/2(TestOk) -> DebStepSelection/1(TestOk), SetNtcSts/3(NtcSts), HwAg1TestOk/1
  AdjStepCalc/3(ParamByte) -> SetNtcSts/2(NtcStInfo)

== system CM670A_HwAg1Meas/HwAg1Meas/HwAg1MeasPer4/HwAgRead/If Action Subsystem1 ==
  Action Port : ActionPort  ActionType=then
  CopyRight2 : Subsystem  Description=|  mask(Copyright Information){none=on}
      | Copyright info block.                                               
      |                                                                     
      | Place copyright information at the top of every subsystem in design.
      mask prompts: none "No parameters"
      mask help: Place copyright information at the top of every subsystem in design.
      mask Display:
      | NxtrConf = 'Nexteer Confidential';
      | 
      | sys = bdroot; %handle for the current model ("system")
      | first = get_param(sys,'Created');
      | first = first(end-3:end);  %year is last four digits
      | 
      | last = get_param(sys,'LastModifiedDate');
      | if isempty(last)
      |     last = datestr(now,'yyyy');
      | else
      |     last = last(end-3:end);
      | end
      | 
      | if strcmp(first,last)
      |     fprintf('%s -- Copyright %s Nexteer',NxtrConf,first)
      | else
      |     fprintf('%s -- %s%s- %s Nexteer',NxtrConf,char(169),first,last)
      | end
  Data Type Conversion : DataTypeConversion  OutDataTypeStr=uint8
  SigQlfr : simulink/Sources/Enumerated Constant  OutDataTypeStr=Enum: SigQlfr1  Value=SigQlfr1.SIGQLFR_PASSD  SampleTime=inf
  Qlfr : Outport
  wires:
  SigQlfr/1 -> Data Type Conversion/1
  Data Type Conversion/1 -> Qlfr/1

== system CM670A_HwAg1Meas/HwAg1Meas/HwAg1MeasPer4/HwAgRead/If Action Subsystem2 ==
  note: Information only:
      |
      | - Hold previous value and skip the step
  Action Port : ActionPort  ActionType=else
  CopyRight2 : Subsystem  Description=|  mask(Copyright Information){none=on}
      | Copyright info block.                                               
      |                                                                     
      | Place copyright information at the top of every subsystem in design.
      mask prompts: none "No parameters"
      mask help: Place copyright information at the top of every subsystem in design.
      mask Display:
      | NxtrConf = 'Nexteer Confidential';
      | 
      | sys = bdroot; %handle for the current model ("system")
      | first = get_param(sys,'Created');
      | first = first(end-3:end);  %year is last four digits
      | 
      | last = get_param(sys,'LastModifiedDate');
      | if isempty(last)
      |     last = datestr(now,'yyyy');
      | else
      |     last = last(end-3:end);
      | end
      | 
      | if strcmp(first,last)
      |     fprintf('%s -- Copyright %s Nexteer',NxtrConf,first)
      | else
      |     fprintf('%s -- %s%s- %s Nexteer',NxtrConf,char(169),first,last)
      | end
  Data Type Conversion : DataTypeConversion  OutDataTypeStr=uint8
  NtcSts1 : simulink/Sources/Enumerated Constant  OutDataTypeStr=Enum: NtcSts1  Value=NtcSts1.NTCSTS_PREFAILD  SampleTime=inf
  TestOk : Outport
  wires:
  NtcSts1/1 -> Data Type Conversion/1
  Data Type Conversion/1 -> TestOk/1
